simulink model "Dummy"  (Simulink 8.4)
settings: Solver=ode45  StartTime=0.0  StopTime=10.0  RelTol=1e-3
undefined symbols (not defined in the file): dummy_facAirPumpRateReq, dummy_facChOverVlvRateReq, dummy_flgInterCoolerOverride, dummy_flgKl50Override, dummy_flgT2tOverride, dummy_rpmFuelPumpMin, dummy_stAirInjReacPumpReq, dummy_StarterReq, dummy_stFuelPumpReq, dummy_stIntercoolerReq, dummy_stMainRelaisReq
settings Model: Creator=YAL9FE  LastModifiedBy=ric9fe
settings DebuggingCC: FcnCallInpInsideContextMsg=EnableAllAsWarning

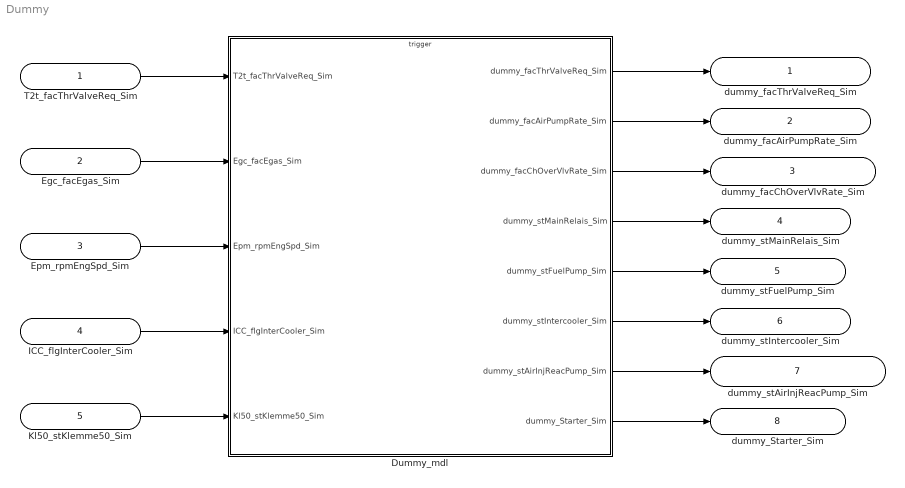
== system Dummy ==
  T2t_facThrValveReq_Sim : Inport
  Egc_facEgas_Sim : Inport  Port=2
  Epm_rpmEngSpd_Sim : Inport  Port=3
  ICC_flgInterCooler_Sim : Inport  Port=4
  Kl50_stKlemme50_Sim : Inport  Port=5
  Dummy_mdl : Subsystem  mask(Functions){}
      mask help: Dummy
      mask Display:
      | image(imread('Dummy.jpg'))
      | port_label('input',1,'T2t_facThrValveReq_Sim')
      | port_label('input',2,'Egc_facEgas_Sim')
      | port_label('input',3,'Epm_rpmEngSpd_Sim')
      | port_label('input',4,'ICC_flgInterCooler_Sim')
      | port_label('input',5,'Kl50_stKlemme50_Sim')
      | port_label('output',1,'dummy_facThrValveReq_Sim')
      | port_label('output',2,'dummy_facAirPumpRate_Sim')
      | port_label('output',3,'dummy_facChOverVlvRate_Sim')
      | port_label('output',4,'dummy_stMainRelais_Sim')
      | port_label('output',5,'dummy_stFuelPump_Sim')
      | port_label('output',6,'dummy_stIntercooler_Sim')
      | port_label('output',7,'dummy_stAirInjReacPump_Sim')
      | port_label('output',8,'dummy_Starter_Sim')
  dummy_facThrValveReq_Sim : Outport
  dummy_facAirPumpRate_Sim : Outport  Port=2
  dummy_facChOverVlvRate_Sim : Outport  Port=3
  dummy_stMainRelais_Sim : Outport  Port=4
  dummy_stFuelPump_Sim : Outport  Port=5
  dummy_stIntercooler_Sim : Outport  Port=6
  dummy_stAirInjReacPump_Sim : Outport  Port=7
  dummy_Starter_Sim : Outport  Port=8
  wires:
  T2t_facThrValveReq_Sim/1 -> Dummy_mdl/1(T2t_facThrValveReq_Sim)
  Egc_facEgas_Sim/1 -> Dummy_mdl/2(Egc_facEgas_Sim)
  Epm_rpmEngSpd_Sim/1 -> Dummy_mdl/3(Epm_rpmEngSpd_Sim)
  ICC_flgInterCooler_Sim/1 -> Dummy_mdl/4(ICC_flgInterCooler_Sim)
  Kl50_stKlemme50_Sim/1 -> Dummy_mdl/5(Kl50_stKlemme50_Sim)
  Dummy_mdl/1(dummy_facThrValveReq_Sim) -> dummy_facThrValveReq_Sim/1
  Dummy_mdl/2(dummy_facAirPumpRate_Sim) -> dummy_facAirPumpRate_Sim/1
  Dummy_mdl/3(dummy_facChOverVlvRate_Sim) -> dummy_facChOverVlvRate_Sim/1
  Dummy_mdl/4(dummy_stMainRelais_Sim) -> dummy_stMainRelais_Sim/1
  Dummy_mdl/5(dummy_stFuelPump_Sim) -> dummy_stFuelPump_Sim/1
  Dummy_mdl/6(dummy_stIntercooler_Sim) -> dummy_stIntercooler_Sim/1
  Dummy_mdl/7(dummy_stAirInjReacPump_Sim) -> dummy_stAirInjReacPump_Sim/1
  Dummy_mdl/8(dummy_Starter_Sim) -> dummy_Starter_Sim/1

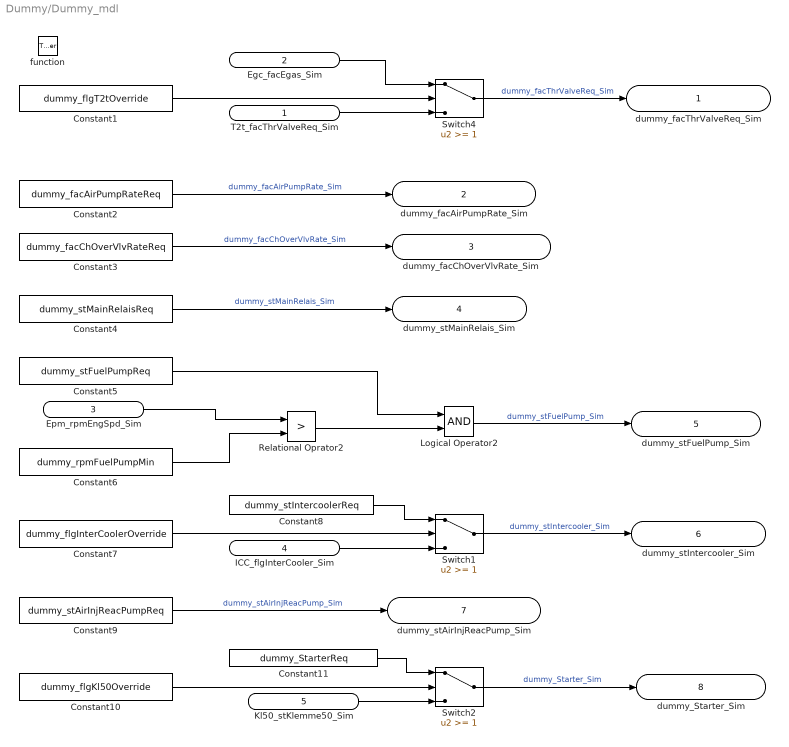
== system Dummy/Dummy_mdl ==
  T2t_facThrValveReq_Sim : Inport
  Egc_facEgas_Sim : Inport  Port=2
  Epm_rpmEngSpd_Sim : Inport  Port=3
  ICC_flgInterCooler_Sim : Inport  Port=4
  Kl50_stKlemme50_Sim : Inport  Port=5
  function : TriggerPort  TriggerType=function-call
  Constant1 : Constant  Value=dummy_flgT2tOverride
  Constant10 : Constant  Value=dummy_flgKl50Override
  Constant11 : Constant  Value=dummy_StarterReq
  Constant2 : Constant  Value=dummy_facAirPumpRateReq
  Constant3 : Constant  Value=dummy_facChOverVlvRateReq
  Constant4 : Constant  Value=dummy_stMainRelaisReq
  Constant5 : Constant  Value=dummy_stFuelPumpReq
  Constant6 : Constant  Value=dummy_rpmFuelPumpMin
  Constant7 : Constant  Value=dummy_flgInterCoolerOverride
  Constant8 : Constant  Value=dummy_stIntercoolerReq
  Constant9 : Constant  Value=dummy_stAirInjReacPumpReq
  Logical Operator2 : Logic  AllPortsSameDT=off  OutDataTypeStr=boolean
  Relational Oprator2 : RelationalOperator  Operator=>  OutDataTypeStr=boolean
  Switch1 : Switch  Threshold=1
  Switch2 : Switch  Threshold=1
  Switch4 : Switch  Threshold=1
  dummy_facThrValveReq_Sim : Outport
  dummy_facAirPumpRate_Sim : Outport  Port=2
  dummy_facChOverVlvRate_Sim : Outport  Port=3
  dummy_stMainRelais_Sim : Outport  Port=4
  dummy_stFuelPump_Sim : Outport  Port=5
  dummy_stIntercooler_Sim : Outport  Port=6
  dummy_stAirInjReacPump_Sim : Outport  Port=7
  dummy_Starter_Sim : Outport  Port=8
  wires:
  Egc_facEgas_Sim/1 -> Switch4/1
  Constant1/1 -> Switch4/2
  T2t_facThrValveReq_Sim/1 -> Switch4/3
  Switch4/1 -> dummy_facThrValveReq_Sim/1  "dummy_facThrValveReq_Sim"
  Constant2/1 -> dummy_facAirPumpRate_Sim/1  "dummy_facAirPumpRate_Sim"
  Constant3/1 -> dummy_facChOverVlvRate_Sim/1  "dummy_facChOverVlvRate_Sim"
  Constant4/1 -> dummy_stMainRelais_Sim/1  "dummy_stMainRelais_Sim"
  Epm_rpmEngSpd_Sim/1 -> Relational Oprator2/1
  Relational Oprator2/1 -> Logical Operator2/2
  Constant5/1 -> Logical Operator2/1
  Logical Operator2/1 -> dummy_stFuelPump_Sim/1  "dummy_stFuelPump_Sim"
  Constant6/1 -> Relational Oprator2/2
  Constant7/1 -> Switch1/2
  Constant8/1 -> Switch1/1
  ICC_flgInterCooler_Sim/1 -> Switch1/3
  Switch1/1 -> dummy_stIntercooler_Sim/1  "dummy_stIntercooler_Sim"
  Constant9/1 -> dummy_stAirInjReacPump_Sim/1  "dummy_stAirInjReacPump_Sim"
  Kl50_stKlemme50_Sim/1 -> Switch2/3
  Constant11/1 -> Switch2/1
  Constant10/1 -> Switch2/2
  Switch2/1 -> dummy_Starter_Sim/1  "dummy_Starter_Sim"
